simulink model "acc_non_eq_v_0_1"  (R2016b)
settings: Solver=VariableStepAuto  StartTime=0.0  StopTime=1800  FixedStep=0.1  RelTol=1e-3
libraries: simulink x1
settings Model: Creator=lanere  LastModifiedBy=lanere

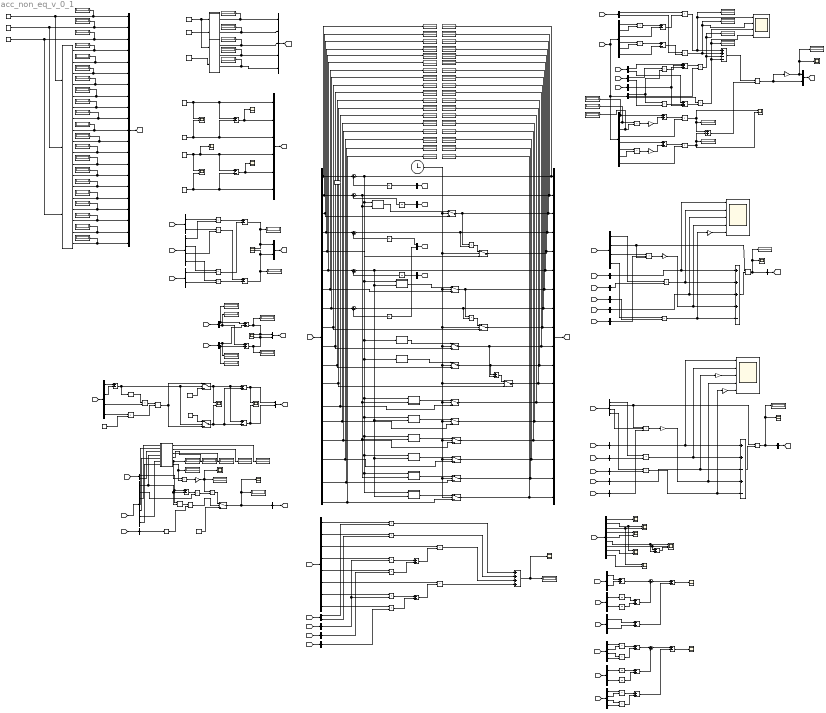
== system acc_non_eq_v_0_1 ==
  note: q_21
  note: Display Center
  note: dh_2dt
  note: dh_1dt
  note: dpdt
  note: m_dot_pt_1 and m_dot_pt_2
  note: m_dot_1 and m_dot_2
  note: Accumulator Inlet Conditions
  note: m_dot_1b and m_dot_2b
  note: mh_dot_1b and mh_dot_2b
  " G_i Display" : Display
  Abs : Abs
  Acc Initial Level : Constant  Value=0.5
  Acc Initial Press : Constant  Value=40.0
  Acc Volume : Constant  Value=64
  Acc Volume Display : Display
  Add{,1..5} (6 alike) : Sum  Inputs=+-
  Add10 : Sum  Inputs=++-
  Add{6..7,11,14..18,20..25} (14 alike) : Sum
  Add12 : Sum  Inputs=++++-
  Add13 : Sum  Inputs=++-+-
  Add19 : Sum  Inputs=++++
  Add8 : Sum  Inputs=++--
  Add9 : Sum  Inputs=+++
  Bus Creator : BusCreator  Inputs=21
  Bus Creator1 : BusCreator  Inputs=5
  Bus Creator10 : BusCreator  Inputs=1
  Bus Creator2 : BusCreator  Inputs=6
  Bus Creator3 : BusCreator  Inputs=18
  Bus Creator{4..6,8} (4 alike) : BusCreator  Inputs=2
  Bus Creator7 : BusCreator  Inputs=1
  Bus Creator9 : BusCreator  Inputs=1
  Bus Selector : BusSelector  OutputSignals=initial_p,initial_h_1,initial_v_1,initial_m_1,initial_vol_1,initial_h_2,initial_v_2,initial_m_2,initial_vol_2,initial_h_f,initial_h_g,initial_r,initial_dvdh_1,initial_dvdh_2,initial_dvdp_1,initial_dvdp_2,initial_t_1,initial_t_2
  Bus Selector1 : BusSelector  OutputSignals=m_dot_1_in,m_dot_1_out,m_dot_2_in,m_dot_2_out
  Bus Selector10 : BusSelector  OutputSignals=t_2_in,v_2_in
  Bus Selector11 : BusSelector  OutputSignals=m_dot_2_in
  Bus Selector12 : BusSelector  OutputSignals=t_1,vol_1,p,v_1,h_1,h_f,r
  Bus Selector13 : BusSelector  OutputSignals=h_g,dvdh_1,dvdh_2
  Bus Selector14 : BusSelector  OutputSignals=mh_dot_1b,mh_dot_2b
  Bus Selector15 : BusSelector  OutputSignals=m_dot_pt_1,m_dot_pt_2
  Bus Selector16 : BusSelector  OutputSignals=q_21
  Bus Selector17 : BusSelector  OutputSignals=dvdp_1,v_1,dvdh_1,m_1,dvdp_2,v_2,dvdh_2,m_2
  Bus Selector18 : BusSelector  OutputSignals=p_dot
  Bus Selector19 : BusSelector  OutputSignals=h_g,m_1,v_1,h_1
  Bus Selector2 : BusSelector  OutputSignals=h_1,h_2
  Bus Selector20 : BusSelector  OutputSignals=mh_dot_1b
  Bus Selector21 : BusSelector  OutputSignals=m_dot_pt_1
  Bus Selector22 : BusSelector  OutputSignals=q_21
  Bus Selector23 : BusSelector  OutputSignals=p_dot_MPA
  Bus Selector24 : BusSelector  OutputSignals=m_dot_1
  Bus Selector25 : BusSelector  OutputSignals=h_dot_1
  Bus Selector26 : BusSelector  OutputSignals=h_g,m_2,v_2,h_2
  Bus Selector27 : BusSelector  OutputSignals=mh_dot_2b
  Bus Selector28 : BusSelector  OutputSignals=m_dot_pt_2
  Bus Selector29 : BusSelector  OutputSignals=q_21
  Bus Selector3 : BusSelector  OutputSignals=h_1_in,h_2_in
  Bus Selector30 : BusSelector  OutputSignals=p_dot_MPA
  Bus Selector31 : BusSelector  OutputSignals=m_dot_2
  Bus Selector32 : BusSelector  OutputSignals=h_dot_2
  Bus Selector33 : BusSelector  OutputSignals=p,h_1,h_2,v_1,v_2,vol_1,vol_2,h_f,h_g
  Bus Selector34 : BusSelector  OutputSignals=v_1,v_2,m_1,dvdp_1,dvdh_1,m_2,dvdp_2,dvdh_2
  Bus Selector35 : BusSelector  OutputSignals=m_dot_1,m_dot_2
  Bus Selector36 : BusSelector  OutputSignals=p_dot_MPA
  Bus Selector37 : BusSelector  OutputSignals=h_dot_1
  Bus Selector38 : BusSelector  OutputSignals=h_dot_2
  Bus Selector39 : BusSelector  OutputSignals=initial_m_1,initial_m_2
  Bus Selector4 : BusSelector  OutputSignals=h_1,h_f,m_1,r
  Bus Selector40 : BusSelector  OutputSignals=m_1,m_2
  Bus Selector41 : BusSelector  OutputSignals=m_dot_1b,m_dot_2b
  Bus Selector42 : BusSelector  OutputSignals=initial_m_1,initial_h_1,initial_m_2,initial_h_2
  Bus Selector43 : BusSelector  OutputSignals=m_1,h_1,m_2,h_2
  Bus Selector44 : BusSelector  OutputSignals=mh_dot_1b,mh_dot_2b
  Bus Selector5 : BusSelector  OutputSignals=m_dot_1b,m_dot_2b
  Bus Selector6 : BusSelector  OutputSignals=m_dot_pt_1,m_dot_pt_2
  Bus Selector7 : BusSelector  OutputSignals=m_dot_1,m_dot_2
  Bus Selector8 : BusSelector  OutputSignals=h_1,dvdh_1,v_1,h_2,dvdh_2,v_2
  Bus Selector9 : BusSelector  OutputSignals=m_dot_1,m_dot_2
  Clock : Clock
  Compare To Zero : simulink/Logic and Bit Operations/Compare To Zero  relop=>  OutDataTypeStr=boolean
  Constant : Constant  Value=0
  Constant1 : Constant  Value=0
  Constant2 : Constant  Value=0
  D_b Display : Display
  Display{,1..16} (17 alike) : Display
  Divide : Product  Inputs=*/
  Divide1 : Product  Inputs=*/
  Divide2 : Product  Inputs=/*
  Divide3 : Product  Inputs=/*
  FW Subcooling : Constant  Value=15.00
  Gain : Gain  Gain=-1
  Gain{1..2,4..5} (4 alike) : Gain  Gain=1000
  Gain3 : Gain  Gain=10
  Gain6 : Gain  Gain=-1
  Gain7 : Gain  Gain=-1
  Initial Level Display : Display
  Initial Press Display : Display
  Initial dvdh_1 Display : Display
      settings: Format=short_e
  Initial dvdh_2 Display : Display
      settings: Format=short_e
  Initial dvdp_1 Display : Display
      settings: Format=short_e
  Initial dvdp_2 Display : Display
      settings: Format=short_e
  Initial h_1 Display : Display
  Initial h_2 Display : Display
  Initial h_f Display : Display
  Initial h_g Display : Display
  Initial m_1 Display : Display
  Initial m_2 Display : Display
      settings: Format=short_e
  Initial r Display : Display
  Initial t_1 Display : Display
  Initial t_2 Display : Display
  Initial v_1 Display : Display
      settings: Format=short_e
  Initial v_2 Display : Display
      settings: Format=short_e
  Initial vol_1 Display : Display
  Initial vol_2 Display : Display
  Initial x Display : Display
  Integrator{,1..8} (9 alike) : Integrator
  Logical Operator : Logic  AllPortsSameDT=off  OutDataTypeStr=boolean
  Product{,1..23,25..26,28..40} (39 alike) : Product
  Product24 : Product  Inputs=3
  Product27 : Product  Inputs=3
  Relational Operator : RelationalOperator  Operator=>  OutDataTypeStr=boolean  RndMeth=Simplest
  SG Pressure : Constant  Value=72.0
  SG Quality : Constant  Value=1.00
  Scope{,1,4..7,16} (7 alike) : Scope  NumInputPorts=2
  Scope{2..3,8..11,13,17..18} (9 alike) : Scope
  Scope12 : Scope  NumInputPorts=5
  Scope14 : Scope  NumInputPorts=5
  Scope15 : Scope  NumInputPorts=4
  Subtract : Sum  Inputs=-+
  Subtract{1..6} (6 alike) : Sum  Inputs=+-
  Sum{,1..6} (7 alike) : Sum  Inputs=|++
  Switch{,1..10,13..14} (13 alike) : Switch  Criteria=u2 ~= 0
  Switch11 : Switch
  Switch12 : Switch
  Switch15 : Switch  Criteria=u2 > Threshold
  Tau : Constant  Value=85.0
  W to KW : Gain  Gain=0.001
  a_i Display : Display
  dvdh_1_0 Display : Display
      settings: Format=short_e
  dvdh_1_f Display : Display
      settings: Format=short_e
  dvdh_2_0 Display : Display
      settings: Format=short_e
  dvdh_2_f Display : Display
      settings: Format=short_e
  dvdp_1_0 Display : Display
      settings: Format=short_e
  dvdp_1_f Display : Display
      settings: Format=short_e
  dvdp_2_0 Display : Display
      settings: Format=short_e
  dvdp_2_f Display : Display
      settings: Format=short_e
  get_dvdh_1 : MATLAB Function  TreatAsAtomicUnit=on
  get_dvdh_2 : MATLAB Function  TreatAsAtomicUnit=on
  get_dvdp_1 : MATLAB Function  TreatAsAtomicUnit=on
  get_dvdp_2 : MATLAB Function  TreatAsAtomicUnit=on
  get_h_f : MATLAB Function  TreatAsAtomicUnit=on
  get_h_g : MATLAB Function  TreatAsAtomicUnit=on
  get_initial_props : MATLAB Function  TreatAsAtomicUnit=on
  get_inlet_cond_1 : MATLAB Function  TreatAsAtomicUnit=on
  get_inlet_cond_2 : MATLAB Function  TreatAsAtomicUnit=on
  get_k_2i_ai : MATLAB Function  TreatAsAtomicUnit=on
  get_t_1 : MATLAB Function  TreatAsAtomicUnit=on
  get_t_2 : MATLAB Function  TreatAsAtomicUnit=on
  get_v_1 : MATLAB Function  TreatAsAtomicUnit=on
  get_v_2 : MATLAB Function  TreatAsAtomicUnit=on
  h_1 vs. h_f : Scope  NumInputPorts=2
  h_1 and h_2 : Scope  NumInputPorts=2
  h_1_0 Display : Display
  h_1_f Display : Display
  h_1_in Display : Display
  h_2 vs. h_g : Scope  NumInputPorts=2
  h_2_0 Display : Display
  h_2_f Display : Display
  h_2_in Display : Display
  h_f_0 Display : Display
  h_f_f Display : Display
  h_g_0 Display : Display
  h_g_f Display : Display
  k_2i Display : Display
  k_2i_ai Scope : Scope
  k_2i_ai_in_kW Display : Display
  m_1_0 Display : Display
      settings: Format=short_e
  m_1_f Display : Display
      settings: Format=short_e
  m_2_0 Display : Display
      settings: Format=short_e
  m_2_f Display : Display
      settings: Format=short_e
  m_dot_1_in : DiscretePulseGenerator  PulseType=Time based  Amplitude=0  Period=60  PulseWidth=50
  m_dot_1_out : DiscretePulseGenerator  PulseType=Time based  Amplitude=0  Period=60  PulseWidth=50  PhaseDelay=30
  m_dot_2_in : DiscretePulseGenerator  PulseType=Time based  Amplitude=2  Period=2800  PulseWidth=25  PhaseDelay=900
  m_dot_2_out : DiscretePulseGenerator  PulseType=Time based  Amplitude=2  Period=2800  PulseWidth=25  PhaseDelay=100
  n Display : Display
  p : Scope
  p_0 Display : Display
  p_f Display : Display
  q_21 Display : Display
      settings: Format=short_e
  q_21 Scope : Scope
  r_0 Display : Display
  r_f Display : Display
  t_1_0 Display : Display
  t_1_f Display : Display
  t_1_in Display : Display
  t_2_0 Display : Display
  t_2_f Display : Display
  t_2_in Display : Display
  term_1 Display : Display
      settings: Format=short_e
  term_2 Display : Display
      settings: Format=short_e
  term_3 Display : Display
      settings: Format=short_e
  term_4 Display : Display
      settings: Format=short_e
  u_2 Display : Display
  v_1 and v_2 : Scope  NumInputPorts=2
  v_1_0 Display : Display
  v_1_f Display : Display
  v_2_0 Display : Display
  v_2_f Display : Display
  v_2_in Display : Display
  vol_1 and vol_2 : Scope  NumInputPorts=3
  vol_1_0 Display : Display
  vol_1_f Display : Display
  vol_2_0 Display : Display
  vol_2_f Display : Display
  wires:
  Acc Initial Level/1 -> Initial Level Display/1, Bus Creator/2, get_initial_props/2(L)  "initial_L"
  get_initial_props/5(m_1) -> Initial m_1 Display/1, Bus Creator/8  "initial_m_1"
  get_initial_props/4(vol_1) -> Initial vol_1 Display/1, Bus Creator/7  "initial_vol_1"
  Acc Volume/1 -> Acc Volume Display/1, Bus Creator/3, get_initial_props/3(V)  "V"
  get_initial_props/2(v_1) -> Initial v_1 Display/1, Bus Creator/5  "initial_v_1"
  get_initial_props/3(t_1) -> Initial t_1 Display/1, Bus Creator/6  "initial_t_1"
  get_initial_props/1(h_1) -> Initial h_1 Display/1, Bus Creator/4  "initial_h_1"
  Acc Initial Press/1 -> Bus Creator/1, Initial Press Display/1, get_initial_props/1(p)  "initial_p"
  get_initial_props/11(x) -> Bus Creator/14, Initial x Display/1  "initial_x"
  get_initial_props/8(t_2) -> Bus Creator/11, Initial t_2 Display/1  "initial_t_2"
  get_initial_props/7(v_2) -> Initial v_2 Display/1, Bus Creator/10  "initial_v_2"
  get_initial_props/10(m_2) -> Bus Creator/13, Initial m_2 Display/1  "initial_m_2"
  get_initial_props/6(h_2) -> Initial h_2 Display/1, Bus Creator/9  "initial_h_2"
  get_initial_props/9(vol_2) -> Bus Creator/12, Initial vol_2 Display/1  "initial_vol_2"
  Bus Creator/1 -> [A]
  SG Quality/1 -> get_inlet_cond_2/2(x)
  SG Pressure/1 -> get_inlet_cond_2/1(p), get_inlet_cond_1/1(p)
  FW Subcooling/1 -> get_inlet_cond_1/2(t_sub)
  get_inlet_cond_1/1(h_1_in) -> h_1_in Display/1, Bus Creator1/1
  get_inlet_cond_1/2(t_1_in) -> t_1_in Display/1, Bus Creator1/2
  get_inlet_cond_2/1(h_2_in) -> Bus Creator1/3, h_2_in Display/1
  get_inlet_cond_2/2(t_2_in) -> Bus Creator1/4, t_2_in Display/1
  [A] -> Bus Selector/1
  m_dot_1_in/1 -> Bus Creator2/1, Add/1, Scope/1  "m_dot_1_in"
  m_dot_1_out/1 -> Bus Creator2/3, Add/2, Scope/2  "m_dot_1_out"
  m_dot_2_in/1 -> Scope1/1, Scope13/1, Add1/1, Bus Creator2/4  "m_dot_2_in"
  m_dot_2_out/1 -> Bus Creator2/6, Add1/2, Scope1/2  "m_dot_2_out"
  Bus Creator1/1 -> [B]
  Add/1 -> Scope2/1, Bus Creator2/2  "m_dot_1b"
  Add1/1 -> Bus Creator2/5, Scope3/1  "m_dot_2b"
  Bus Creator2/1 -> [C]
  get_initial_props/12(h_f) -> Initial h_f Display/1, Bus Creator/15  "initial_h_f"
  get_initial_props/13(h_g) -> Initial h_g Display/1, Bus Creator/16  "initial_h_g"
  get_initial_props/14(r) -> Initial r Display/1, Bus Creator/17  "initial_r"
  Bus Selector/1 -> p_0 Display/1, Sum/1  "<initial_p>"
  Bus Selector/2 -> h_1_0 Display/1, Sum1/1  "<initial_h_1>"
  Bus Selector/4 -> m_1_0 Display/1, Sum2/1  "<initial_m_1>"
  Bus Selector/6 -> h_2_0 Display/1, Sum3/1  "<initial_h_2>"
  Bus Selector/8 -> m_2_0 Display/1, Sum4/1  "<initial_m_2>"
  Sum/1 -> p_f Display/1, Bus Creator3/1, get_dvdh_1/1(p), get_dvdh_2/1(p), get_dvdp_1/1(p), get_t_2/1(p), get_t_1/1(p), get_dvdp_2/1(p), get_h_g/1(p), get_h_f/1(p), get_v_2/1(p), get_v_1/1(p)  "p"
  Sum1/1 -> h_1_f Display/1, Bus Creator3/2, get_dvdh_1/2(h), get_t_1/2(h), get_dvdp_1/2(h), get_v_1/2(h)  "h_1"
  Sum2/1 -> m_1_f Display/1, Bus Creator3/4, Product4/2  "m_1"
  Sum3/1 -> h_2_f Display/1, Bus Creator3/6, get_t_2/2(h), get_dvdp_2/2(h), get_dvdh_2/2(h), get_v_2/2(h)  "h_2"
  Sum4/1 -> m_2_f Display/1, Bus Creator3/8, Product5/2  "m_2"
  Bus Creator3/1 -> [D]
  [C] -> Bus Selector1/1
  [D] -> Bus Selector2/1
  [B] -> Bus Selector3/1
  Bus Selector1/1 -> Product/2  "<m_dot_1_in>"
  Bus Selector3/1 -> Product/1  "<h_1_in>"
  Bus Selector3/2 -> Product1/1  "<h_2_in>"
  Bus Selector1/3 -> Product1/2  "<m_dot_2_in>"
  Bus Selector1/2 -> Product2/1  "<m_dot_1_out>"
  Bus Selector1/4 -> Product3/1  "<m_dot_2_out>"
  Bus Selector2/1 -> Product2/2  "<h_1>"
  Bus Selector2/2 -> Product3/2  "<h_2>"
  Product/1 -> Add2/1  "mh_dot_1_in"
  Product1/1 -> Add3/1  "mh_dot_2_in"
  Product2/1 -> Add2/2  "mh_dot_1_out"
  Product3/1 -> Add3/2  "mh_dot_2_out"
  Bus Creator4/1 -> [E]
  [C] -> Bus Selector5/1
  Add2/1 -> Display6/1, Scope4/1, Bus Creator4/1  "mh_dot_1b"
  Add3/1 -> Display7/1, Scope4/2, Bus Creator4/2  "mh_dot_2b"
  Switch/1 -> v_1_f Display/1, Bus Creator3/3, Product4/1  "v_1"
  get_v_1/1(v_1) -> Switch/1
  Switch1/1 -> v_2_f Display/1, Bus Creator3/7, Product5/1  "v_2"
  get_v_2/1(v_2) -> Switch1/1
  Bus Selector/7 -> v_2_0 Display/1, Switch1/3  "<initial_v_2>"
  Bus Selector/3 -> Switch/3, v_1_0 Display/1  "<initial_v_1>"
  Clock/1 -> Switch2/2, Switch10/2, Switch13/2, Switch14/2, Switch9/2, Switch8/2, Switch7/2, Switch6/2, Switch5/2, Switch4/2, Switch3/2, Switch1/2, Switch/2
  Switch2/1 -> vol_1_f Display/1, Bus Creator3/5  "vol_1"
  Switch3/1 -> vol_2_f Display/1, Bus Creator3/9  "vol_2"
  Product4/1 -> Switch2/1
  Product5/1 -> Switch3/1
  Bus Selector/5 -> vol_1_0 Display/1, Switch2/3  "<initial_vol_1>"
  Bus Selector/9 -> vol_2_0 Display/1, Switch3/3  "<initial_vol_2>"
  Bus Selector/10 -> h_f_0 Display/1, Switch4/3  "<initial_h_f>"
  Switch4/1 -> Add4/2, h_f_f Display/1, Bus Creator3/10  "h_f"
  Switch5/1 -> Add4/1, h_g_f Display/1, Bus Creator3/11  "h_g"
  Switch6/1 -> r_f Display/1, Bus Creator3/12  "r"
  Bus Selector/11 -> h_g_0 Display/1, Switch5/3  "<initial_h_g>"
  Bus Selector/12 -> Switch6/3, r_0 Display/1  "<initial_r>"
  Add4/1 -> Switch6/1
  get_h_f/1(h_f) -> Switch4/1
  get_h_g/1(h_g) -> Switch5/1
  get_initial_props/15(dvdh_1) -> Initial dvdh_1 Display/1, Bus Creator/18  "initial_dvdh_1"
  get_initial_props/16(dvdp_1) -> Initial dvdp_1 Display/1, Bus Creator/19  "initial_dvdp_1"
  get_initial_props/17(dvdh_2) -> Initial dvdh_2 Display/1, Bus Creator/20  "initial_dvdh_2"
  get_initial_props/18(dvdp_2) -> Initial dvdp_2 Display/1, Bus Creator/21  "initial_dvdp_2"
  Bus Selector/13 -> dvdh_1_0 Display/1, Switch7/3  "<initial_dvdh_1>"
  Switch8/1 -> dvdh_2_f Display/1, Bus Creator3/14  "dvdh_2"
  Switch9/1 -> dvdp_1_f Display/1, Bus Creator3/15  "dvdp_1"
  Switch10/1 -> dvdp_2_f Display/1, Bus Creator3/16  "dvdp_2"
  Bus Selector/16 -> dvdp_2_0 Display/1, Switch10/3  "<initial_dvdp_2>"
  get_dvdh_1/1(dvdh_1) -> Switch7/1
  get_dvdh_2/1(dvdh_2) -> Switch8/1
  get_dvdp_1/1(dvdp_1) -> Switch9/1
  get_dvdp_2/1(dvdp_2) -> Switch10/1
  Switch7/1 -> dvdh_1_f Display/1, Bus Creator3/13  "dvdh_1"
  Bus Selector/14 -> dvdh_2_0 Display/1, Switch8/3  "<initial_dvdh_2>"
  Bus Selector/15 -> dvdp_1_0 Display/1, Switch9/3  "<initial_dvdp_1>"
  [D] -> Bus Selector4/1
  Bus Selector4/1 -> Add5/1  "<h_1>"
  Bus Selector4/2 -> Add5/2  "<h_f>"
  Add5/1 -> Switch12/2, Switch11/2, Abs/1
  Bus Selector4/3 -> Product6/2  "<m_1>"
  Bus Selector4/4 -> Product7/1  "<r>"
  Abs/1 -> Product6/1
  Tau/1 -> Product7/2
  Product6/1 -> Divide/1
  Product7/1 -> Divide/2
  Constant/1 -> Switch12/1
  Constant1/1 -> Switch11/3
  Divide/1 -> Switch12/3, Switch11/1
  Switch11/1 -> Subtract1/1, Subtract/1, Scope6/1  "m_e"
  Switch12/1 -> Subtract1/2, Subtract/2, Scope6/2  "m_c"
  Subtract/1 -> Scope7/1, Bus Creator5/1  "m_dot_pt_1"
  Subtract1/1 -> Scope7/2, Bus Creator5/2  "m_dot_pt_2"
  Bus Creator5/1 -> [F]
  [F] -> Bus Selector6/1
  Bus Selector5/1 -> Display2/1, Add6/1  "<m_dot_1b>"
  Bus Selector6/1 -> Display4/1, Add6/2  "<m_dot_pt_1>"
  Bus Selector6/2 -> Display5/1, Add7/2  "<m_dot_pt_2>"
  Bus Selector5/2 -> Display3/1, Add7/1  "<m_dot_2b>"
  Add6/1 -> Display/1, Bus Creator6/1, Scope5/1  "m_dot_1"
  Add7/1 -> Display1/1, Scope5/2, Bus Creator6/2  "m_dot_2"
  Bus Creator6/1 -> [G]
  [G] -> Bus Selector7/1
  Bus Selector7/1 -> Integrator/1  "<m_dot_1>"
  Integrator/1 -> Sum2/2
  Bus Selector7/2 -> Integrator1/1  "<m_dot_2>"
  Integrator1/1 -> Sum4/2
  [D] -> Bus Selector17/1, Bus Selector13/1, Bus Selector8/1
  [G] -> Bus Selector9/1
  Bus Selector8/1 -> Product8/1  "<h_1>"
  Bus Selector8/2 -> Product8/2  "<dvdh_1>"
  Product8/1 -> Subtract2/1
  Bus Selector8/3 -> Subtract2/2  "<v_1>"
  Subtract2/1 -> Product9/2
  Bus Selector9/1 -> Product9/1  "<m_dot_1>"
  Product9/1 -> Scope15/1, term_1 Display/1, Add8/1  "term_1"
  Bus Selector8/4 -> Product10/1  "<h_2>"
  Bus Selector8/5 -> Product10/2  "<dvdh_2>"
  Product10/1 -> Subtract3/1
  Bus Selector8/6 -> Subtract3/2  "<v_2>"
  Subtract3/1 -> Product11/2
  Bus Selector9/2 -> Product11/1  "<m_dot_2>"
  Product11/1 -> Add8/2, Scope15/2, term_2 Display/1  "term_2"
  [B] -> Bus Selector10/1
  [C] -> Bus Selector11/1
  [D] -> Bus Selector12/1
  Switch13/1 -> t_1_f Display/1, Bus Creator3/17  "t_1"
  Switch14/1 -> t_2_f Display/1, Bus Creator3/18  "t_2"
  Bus Selector/18 -> t_2_0 Display/1, Switch14/3  "<initial_t_2>"
  Bus Selector/17 -> t_1_0 Display/1, Switch13/3  "<initial_t_1>"
  get_t_2/1(t_2) -> Switch14/1
  get_t_1/1(t_1) -> Switch13/1
  Bus Selector10/1 -> Subtract4/1, Relational Operator/1  "<t_2_in>"
  Bus Selector11/1 -> Compare To Zero/1  "<m_dot_2_in>"
  Bus Selector12/1 -> get_k_2i_ai/4(t_1), Relational Operator/2, Subtract4/2  "<t_1>"
  Constant2/1 -> Switch15/3
  Subtract4/1 -> Product12/1
  Bus Selector12/2 -> Product12/2  "<vol_1>"
  Product21/1 -> Switch15/1
  Relational Operator/1 -> Logical Operator/1
  Compare To Zero/1 -> Logical Operator/2
  Logical Operator/1 -> Switch15/2
  Switch15/1 -> Bus Creator7/1, q_21 Scope/1, q_21 Display/1  "q_21"
  Bus Creator7/1 -> [H]
  [E] -> Bus Selector14/1
  [F] -> Bus Selector15/1
  Bus Selector15/1 -> Product13/1  "<m_dot_pt_1>"
  Bus Selector15/2 -> Product15/2  "<m_dot_pt_2>"
  Bus Selector14/1 -> Add9/1  "<mh_dot_1b>"
  Bus Selector14/2 -> Add10/1  "<mh_dot_2b>"
  Bus Selector13/1 -> Product15/1, Product13/2  "<h_g>"
  [H] -> Bus Selector16/1
  Bus Selector16/1 -> Add10/3, Add9/3  "<q_21>"
  Product13/1 -> Add9/2
  Add9/1 -> Product14/1
  Bus Selector13/2 -> Product14/2  "<dvdh_1>"
  Product14/1 -> Scope15/3, term_3 Display/1, Add8/3  "term_3"
  Product15/1 -> Add10/2
  Add10/1 -> Product16/2
  Bus Selector13/3 -> Product16/1  "<dvdh_2>"
  Product16/1 -> Add8/4, Scope15/4, term_4 Display/1  "term_4"
  Bus Selector17/1 -> Add14/1, Display10/1  "<dvdp_1>"
  Bus Selector17/2 -> Display11/1, Product17/1  "<v_1>"
  Bus Selector17/3 -> Display12/1, Product17/2  "<dvdh_1>"
  Product17/1 -> Gain1/1
  Gain1/1 -> Add14/2
  Add14/1 -> Product19/1
  Bus Selector17/4 -> Product19/2  "<m_1>"
  Bus Selector17/6 -> Product20/1  "<v_2>"
  Bus Selector17/7 -> Product20/2  "<dvdh_2>"
  Product20/1 -> Gain2/1
  Gain2/1 -> Add15/2
  Bus Selector17/5 -> Add15/1  "<dvdp_2>"
  Add15/1 -> Product22/1
  Bus Selector17/8 -> Product22/2  "<m_2>"
  Product19/1 -> Scope16/1, Display8/1, Add11/1  "term_5"
  Product22/1 -> Scope16/2, Display9/1, Add11/2  "term_6"
  Add8/1 -> Divide1/1
  Add11/1 -> Divide1/2
  Divide1/1 -> Gain3/1, Bus Creator8/2  "p_dot_MPA"
  Bus Creator8/1 -> [I]
  [I] -> Bus Selector18/1
  Bus Selector18/1 -> Integrator2/1  "<p_dot>"
  Integrator2/1 -> Sum/2
  Gain3/1 -> Display14/1, Scope8/1, Bus Creator8/1  "p_dot"
  [D] -> Bus Selector19/1
  [E] -> Bus Selector20/1
  [F] -> Bus Selector21/1
  [H] -> Bus Selector22/1
  [I] -> Bus Selector23/1
  [G] -> Bus Selector24/1
  Bus Selector20/1 -> Scope14/1, Add12/1  "<mh_dot_1b>"
  Bus Selector21/1 -> Product23/2  "<m_dot_pt_1>"
  Bus Selector19/1 -> Product23/1  "<h_g>"
  Bus Selector19/3 -> Product24/1  "<v_1>"
  Bus Selector19/4 -> Product25/1  "<h_1>"
  Bus Selector23/1 -> Product24/2  "<p_dot_MPA>"
  Bus Selector19/2 -> Product24/3, Divide2/1  "<m_1>"
  Product24/1 -> Gain4/1
  Bus Selector22/1 -> Scope14/3, Add12/3  "<q_21>"
  Bus Selector24/1 -> Product25/2  "<m_dot_1>"
  Gain4/1 -> Scope14/4, Add12/4  "m_1 v_1 dpdt"
  Product25/1 -> Add12/5, Gain7/1
  Product23/1 -> Scope14/2, Add12/2  "m_dot_pt_1 h_g"
  Add12/1 -> Divide2/2
  Divide2/1 -> Display13/1, Scope9/1, Bus Creator9/1  "h_dot_1"
  Bus Creator9/1 -> [J]
  [J] -> Bus Selector25/1
  Bus Selector25/1 -> Integrator3/1  "<h_dot_1>"
  Integrator3/1 -> Sum1/2
  [D] -> Bus Selector26/1
  [E] -> Bus Selector27/1
  [F] -> Bus Selector28/1
  [H] -> Bus Selector29/1
  [I] -> Bus Selector30/1
  [G] -> Bus Selector31/1
  Bus Selector27/1 -> Scope12/1, Add13/1  "<mh_dot_2b>"
  Bus Selector28/1 -> Product26/2  "<m_dot_pt_2>"
  Bus Selector26/1 -> Product26/1  "<h_g>"
  Bus Selector26/3 -> Product27/2  "<v_2>"
  Bus Selector26/4 -> Product28/1  "<h_2>"
  Bus Selector30/1 -> Product27/3  "<p_dot_MPA>"
  Bus Selector26/2 -> Product27/1, Divide3/1  "<m_2>"
  Product27/1 -> Gain5/1
  Bus Selector29/1 -> Gain/1, Add13/3  "<q_21>"
  Bus Selector31/1 -> Product28/2  "<m_dot_2>"
  Gain5/1 -> Scope12/4, Add13/4  "m_2 v_2 dpdt"
  Product28/1 -> Gain6/1, Add13/5
  Product26/1 -> Scope12/2, Add13/2  "m_dot_pt_2 h_g"
  Add13/1 -> Divide3/2
  Divide3/1 -> Bus Creator10/1, Scope10/1, Display15/1  "h_dot_2"
  Bus Creator10/1 -> [K]
  [K] -> Bus Selector32/1
  Bus Selector32/1 -> Integrator4/1  "<h_dot_2>"
  Integrator4/1 -> Sum3/2
  [D] -> Bus Selector33/1
  Bus Selector33/1 -> p/1  "<p>"
  Bus Selector33/2 -> h_1 vs. h_f/1, h_1 and h_2/1  "<h_1>"
  Bus Selector33/3 -> h_2 vs. h_g/1, h_1 and h_2/2  "<h_2>"
  Bus Selector33/4 -> v_1 and v_2/1  "<v_1>"
  Bus Selector33/5 -> v_1 and v_2/2  "<v_2>"
  Bus Selector33/6 -> Add16/2, vol_1 and vol_2/1  "<vol_1>"
  Bus Selector33/7 -> vol_1 and vol_2/2, Add16/1  "<vol_2>"
  Bus Selector33/8 -> h_1 vs. h_f/2  "<h_f>"
  Bus Selector33/9 -> h_2 vs. h_g/2  "<h_g>"
  Add16/1 -> vol_1 and vol_2/3  "vol_total"
  get_inlet_cond_2/3(v_2_in) -> v_2_in Display/1, Bus Creator1/5
  Bus Selector10/2 -> get_k_2i_ai/3(v_2)  "<v_2_in>"
  Bus Selector12/3 -> get_k_2i_ai/1(p)  "<p>"
  Bus Selector12/4 -> get_k_2i_ai/2(v_1)  "<v_1>"
  get_k_2i_ai/1(u_2) -> u_2 Display/1  "u_2_in"
  get_k_2i_ai/2(D_b) -> D_b Display/1  "D_b"
  Bus Selector12/5 -> get_k_2i_ai/5(h_1)  "<h_1>"
  Bus Selector12/6 -> get_k_2i_ai/6(h_f)  "<h_f>"
  Bus Selector12/7 -> get_k_2i_ai/7(r)  "<r>"
  get_k_2i_ai/3(G_i) -> " G_i Display"/1
  get_k_2i_ai/4(n) -> n Display/1
  get_k_2i_ai/5(a_i) -> Product18/1, a_i Display/1
  get_k_2i_ai/6(k_2i) -> k_2i Display/1, Product18/2
  Product12/1 -> Product21/2
  Product18/1 -> W to KW/1
  W to KW/1 -> k_2i_ai Scope/1, k_2i_ai_in_kW Display/1, Product21/1
  [D] -> Bus Selector34/1
  [G] -> Bus Selector35/1
  [I] -> Bus Selector36/1
  [J] -> Bus Selector37/1
  [K] -> Bus Selector38/1
  Bus Selector34/1 -> Product29/1  "<v_1>"
  Bus Selector35/1 -> Product29/2  "<m_dot_1>"
  Bus Selector34/2 -> Product30/1  "<v_2>"
  Bus Selector35/2 -> Product30/2  "<m_dot_2>"
  Bus Selector36/1 -> Product35/2, Product31/2  "<p_dot_MPA>"
  Bus Selector37/1 -> Product32/2  "<h_dot_1>"
  Bus Selector34/4 -> Product31/1  "<dvdp_1>"
  Bus Selector34/5 -> Product32/1  "<dvdh_1>"
  Product31/1 -> Add17/1
  Product32/1 -> Add17/2
  Bus Selector34/3 -> Product33/1  "<m_1>"
  Add17/1 -> Product33/2
  Bus Selector34/6 -> Product34/1  "<m_2>"
  Bus Selector34/7 -> Product35/1  "<dvdp_2>"
  Bus Selector34/8 -> Product36/1  "<dvdh_2>"
  Bus Selector38/1 -> Product36/2  "<h_dot_2>"
  Product35/1 -> Add18/1
  Product36/1 -> Add18/2
  Add18/1 -> Product34/2
  Product29/1 -> Add19/1
  Product33/1 -> Add19/3
  Product34/1 -> Add19/4
  Product30/1 -> Add19/2
  Add19/1 -> Scope11/1, Display16/1
  Gain/1 -> Scope12/3  "q_21"
  Gain6/1 -> Scope12/5  "h_2 m_dot_2"
  Gain7/1 -> Scope14/5  "m_dot_1 h_1"
  [A] -> Bus Selector39/1
  [D] -> Bus Selector40/1
  [C] -> Bus Selector41/1
  Bus Selector39/1 -> Add20/1  "<initial_m_1>"
  Bus Selector41/1 -> Integrator5/1  "<m_dot_1b>"
  Bus Selector41/2 -> Integrator6/1  "<m_dot_2b>"
  Bus Selector39/2 -> Add20/2  "<initial_m_2>"
  Add20/1 -> Sum5/1
  Integrator5/1 -> Add21/1
  Integrator6/1 -> Add21/2
  Add21/1 -> Sum5/2
  Sum5/1 -> Subtract5/1
  Bus Selector40/1 -> Add22/1  "<m_1>"
  Bus Selector40/2 -> Add22/2  "<m_2>"
  Add22/1 -> Subtract5/2
  Subtract5/1 -> Scope17/1  "m_defect"
  [A] -> Bus Selector42/1
  Bus Selector42/1 -> Product37/1  "<initial_m_1>"
  Bus Selector42/3 -> Product38/1  "<initial_m_2>"
  Bus Selector42/2 -> Product37/2  "<initial_h_1>"
  Bus Selector42/4 -> Product38/2  "<initial_h_2>"
  Product37/1 -> Add23/1
  Product38/1 -> Add23/2
  [D] -> Bus Selector43/1
  Bus Selector43/1 -> Product39/1  "<m_1>"
  Bus Selector43/3 -> Product40/1  "<m_2>"
  Bus Selector43/2 -> Product39/2  "<h_1>"
  Bus Selector43/4 -> Product40/2  "<h_2>"
  [E] -> Bus Selector44/1
  Bus Selector44/1 -> Integrator7/1  "<mh_dot_1b>"
  Bus Selector44/2 -> Integrator8/1  "<mh_dot_2b>"
  Integrator7/1 -> Add24/1
  Integrator8/1 -> Add24/2
  Add23/1 -> Sum6/1
  Add24/1 -> Sum6/2
  Product39/1 -> Add25/1
  Product40/1 -> Add25/2
  Sum6/1 -> Subtract6/1  "H_calc"
  Add25/1 -> Subtract6/2  "H_act"
  Subtract6/1 -> Scope18/1  "H_defect"

== matlab function acc_non_eq_v_0_1/get_inlet_cond_2 ==
  data: p input; h_2_in output; x input; t_2_in output; v_2_in output
function [h_2_in, t_2_in, v_2_in] = inlet_cond_2(p, x)
coder.extrinsic('XSteam');
h_2_in = 0.0;
t_2_in = 0.0;
v_2_in = 0.0;
v_f = 0.0;
v_g = 0.0;
h_2_in = XSteam('h_px', p, x);
t_2_in = XSteam('Tsat_p', p);
v_f = XSteam('vL_p', p);
v_g = XSteam('vV_p', p);
v_2_in = v_f + x * v_g;

== matlab function acc_non_eq_v_0_1/get_initial_props ==
  data: p input; h_1 output; L input; v_1 output; t_1 output; vol_1 output; m_1 output; h_2 output; v_2 output; t_2 output; vol_2 output; m_2 output; V input; x output; h_f output; h_g output; r output; dvdh_1 output; dvdp_1 output; dvdh_2 output; dvdp_2 output
function [h_1, v_1, t_1, vol_1, m_1, h_2, v_2, t_2, vol_2, m_2, x, h_f, h_g, r, dvdh_1, dvdp_1, dvdh_2, dvdp_2] = init_props(p, L, V)
coder.extrinsic('XSteam');
coder.extrinsic('IAPWS_IF97');
EPSILON = 0.02;
MPA_PER_BAR = 0.1;
h_1 = 0.0;
v_1 = 0.0;
t_1 = 0.0;
vol_1 = 0.0;
m_1 = 0.0;
h_2 = 0.0;
v_2 = 0.0;
t_2 = 0.0;
vol_2 = 0.0;
m_2 = 0.0;
x = 0.0;
h_f = 0.0;
h_g = 0.0;
r = 0.0;
dvdh_1 = 0.0;
dvdp_1 = 0.0;
dvdh_2 = 0.0;
dvdp_2 = 0.0;
t_1 = XSteam('Tsat_p', p);
t_2 = t_1;
t_1 = t_1 - EPSILON;
t_2 = t_2 + EPSILON;
h_1 = XSteam('h_pT', p, t_1);
h_2 = XSteam('h_pT', p, t_2);
v_1 = XSteam('v_ph', p, h_1);
v_2 = XSteam('v_ph', p, h_2);
vol_1 = V * L;
vol_2 = V - vol_1;
m_1 = vol_1 / v_1;
m_2 = vol_2 / v_2;
x = m_2 / (m_1 + m_2);
h_f = XSteam('hL_p', p);
h_g = XSteam('hV_p', p);
r = h_g - h_f;
dvdh_1 = IAPWS_IF97('dvdh_ph', p * MPA_PER_BAR, h_1);
dvdp_1 = IAPWS_IF97('dvdp_ph', p * MPA_PER_BAR, h_1);
dvdh_2 = IAPWS_IF97('dvdh_ph', p * MPA_PER_BAR, h_2);
dvdp_2 = IAPWS_IF97('dvdp_ph', p * MPA_PER_BAR, h_2);

== matlab function acc_non_eq_v_0_1/get_inlet_cond_1 ==
  data: p input; h_1_in output; t_sub input; t_1_in output
function [h_1_in, t_1_in] = inlet_cond_1(p, t_sub)
coder.extrinsic('XSteam');
h_1_in = 0.0;
t_1_in = 0.0;
t_1_in = XSteam('Tsat_p', p);
t_1_in = t_1_in - t_sub;
h_1_in = XSteam('h_pT', p, t_1_in);

== matlab function acc_non_eq_v_0_1/get_v_1 ==
  data: p input; v_1 output; h input
function v_1 = v_ph(p, h)
coder.extrinsic('XSteam');
v_1 = 0.0;
v_1 = XSteam('v_ph', p, h);

== matlab function acc_non_eq_v_0_1/get_v_2 ==
  data: p input; v_2 output; h input
function v_2 = v_ph(p, h)
coder.extrinsic('XSteam');
v_2 = 0.0;
v_2 = XSteam('v_ph', p, h);

== matlab function acc_non_eq_v_0_1/get_h_f ==
  data: p input; h_f output
function h_f = hL_p(p)
coder.extrinsic('XSteam');
h_f = 0.0;
h_f = XSteam('hL_p', p);

== matlab function acc_non_eq_v_0_1/get_h_g ==
  data: p input; h_g output
function h_g = hV_p(p)
coder.extrinsic('XSteam');
h_g = 0.0;
h_g = XSteam('hV_p', p);

== matlab function acc_non_eq_v_0_1/get_dvdh_1 ==
  data: p input; dvdh_1 output; h input
function dvdh_1 = dvdh_ph(p, h)
coder.extrinsic('IAPWS_IF97');
MPA_PER_BAR = 0.1;
dvdh_1 = 0.0;
dvdh_1 = IAPWS_IF97('dvdh_ph', p * MPA_PER_BAR, h);

== matlab function acc_non_eq_v_0_1/get_dvdh_2 ==
  data: p input; dvdh_2 output; h input
function dvdh_2 = dvdh_ph(p, h)
coder.extrinsic('IAPWS_IF97');
MPA_PER_BAR = 0.1;
dvdh_2 = 0.0;
dvdh_2 = IAPWS_IF97('dvdh_ph', p * MPA_PER_BAR, h);

== matlab function acc_non_eq_v_0_1/get_dvdp_1 ==
  data: p input; dvdp_1 output; h input
function dvdp_1 = dvdp_ph(p, h)
coder.extrinsic('IAPWS_IF97');
MPA_PER_BAR = 0.1;
dvdp_1 = 0.0;
dvdp_1 = IAPWS_IF97('dvdp_ph', p * MPA_PER_BAR, h);

== matlab function acc_non_eq_v_0_1/get_dvdp_2 ==
  data: p input; dvdp_2 output; h input
function dvdp_2 = dvdp_ph(p, h)
coder.extrinsic('IAPWS_IF97');
MPA_PER_BAR = 0.1;
dvdp_2 = 0.0;
dvdp_2 = IAPWS_IF97('dvdp_ph', p * MPA_PER_BAR, h);

== matlab function acc_non_eq_v_0_1/get_t_1 ==
  data: p input; t_1 output; h input
function t_1 = T_ph(p, h)
coder.extrinsic('XSteam');
h_f = 0.0;
t_1 = 0.0;
h_f = XSteam('hL_p', p);
if(h < h_f)
    t_1 = XSteam('T_ph', p, h);
else
    t_1 = XSteam('Tsat_p', p);
end

== matlab function acc_non_eq_v_0_1/get_t_2 ==
  data: p input; t_2 output; h input
function t_2 = T_ph(p, h)
coder.extrinsic('XSteam');
h_g = 0.0;
t_2 = 0.0;
h_g = XSteam('hV_p', p);
if(h > h_g)
    t_2 = XSteam('T_ph', p, h);
else
    t_2 = XSteam('Tsat_p', p);
end

== matlab function acc_non_eq_v_0_1/get_k_2i_ai ==
  data: p input; u_2 output; v_1 input; v_2 input; t_1 input; D_b output; h_1 input; h_f input; r input; G_i output; n output; a_i output; k_2i output
function [u_2, D_b, G_i, n, a_i, k_2i]= k_2i_a_i(p, v_1, v_2, t_1, h_1, h_f, r)
coder.extrinsic('XSteam');
rho_1 = 0.0;
rho_2 = 0.0;
st = 0.0;
u_2 = 0.0;
D_b = 0.0;
G_i = 0.0;
n = 0.0;
a_i = 0.0;
tcv_2 = 0.0;
k_2i = 0.0;
g = 9.8;
W_e_cr = 1.24;
k_B = 1.38064852e-23;
rho_1 = 1 / v_1;
rho_2 = 1 / v_2;
st = XSteam('st_p', p);
u_2 = 1.4 * (st * g * (rho_1 - rho_2) / (rho_1^2))^(1/4);
D_b = W_e_cr * st / (rho_1 * (u_2^2));
G_i  = 16 * pi * (st^3) / ((3 * k_B * t_1 * r^2 * ((h_1 / h_f) - 1)^2) * rho_1^2);
G_i = G_i / 1e6;
n = 10^(6.8 - 0.15 * log(G_i));
a_i = n * 4 * pi * (D_b / 2)^2;
tcv_2 = XSteam('tcv_p', p);
k_2i = 16 * tcv_2 / D_b;
